simulink model "HCU_V2_Driver"  (R2023b)
settings: Solver=FixedStepAuto  StartTime=0  StopTime=2474  FixedStep=0.001  RelTol=1e-3
undefined symbols (not defined in the file or in its folder): DiscIntNeverNeededParam
libraries: autolibshared x1, slpidlib x1
settings Model: Creator=volos  LastModifiedBy=volos
settings OptimizationCC: DefaultParameterBehavior=Inlined  EnhancedBackFolding=on  PassReuseOutputArgsAs=Individual arguments  ZeroExternalMemoryAtStartup=off  ZeroInternalMemoryAtStartup=off  OptimizeBlockOrder=speed  DifferentSizesBufferReuse=on  OptimizationCustomize=off  EfficientTunableParamExpr=on
settings DebuggingCC: ParameterTunabilityLossMsg=error
settings SFSimCC: MATLABDynamicMemAlloc=off
settings RTWCC: Description=Embedded Coder  SystemTargetFile=ert.tlc  TemplateMakefile=ert_default_tmf  TargetLang=C++
settings CodeAppCC: ForceParamTrailComments=on  IgnoreCustomStorageClasses=off  OperatorAnnotations=on  SimulinkDataObjDesc=on  SFDataObjDesc=on  InsertBlockDesc=on
settings ERTTargetCC: TargetLangStandard=C++11 (ISO)  GenerateSampleERTMain=on  CodeInterfacePackaging=C++ class  InlinedParameterPlacement=NonHierarchical  RootIOFormat=Structure reference  ERTCustomFileTemplate=example_file_process.tlc

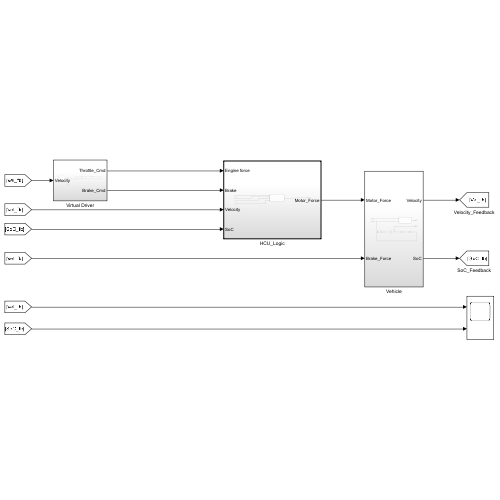
[thumbnail: Simulink's stored preview of the top-level diagram]
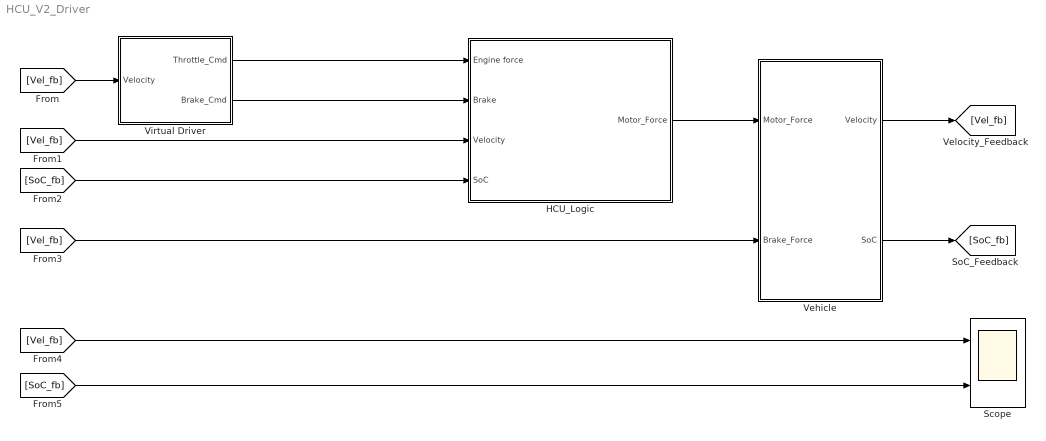
== system HCU_V2_Driver ==
  HCU_Logic : Subsystem  TreatAsAtomicUnit=on
  Scope : Scope  NumInputPorts=2
  Vehicle : Subsystem
  Virtual Driver : Subsystem
  wires:
  Virtual Driver/1(Throttle_Cmd) -> HCU_Logic/1(Engine force)
  Virtual Driver/2(Brake_Cmd) -> HCU_Logic/2(Brake)
  Vehicle/2(SoC) -> [SoC_fb]
  Vehicle/1(Velocity) -> [Vel_fb]
  HCU_Logic/1(Motor_Force) -> Vehicle/1(Motor_Force)
  [Vel_fb] -> Virtual Driver/1(Velocity)
  [Vel_fb] -> HCU_Logic/3(Velocity)
  [SoC_fb] -> HCU_Logic/4(SoC)
  [Vel_fb] -> Vehicle/2(Brake_Force)
  [Vel_fb] -> Scope/1
  [SoC_fb] -> Scope/2

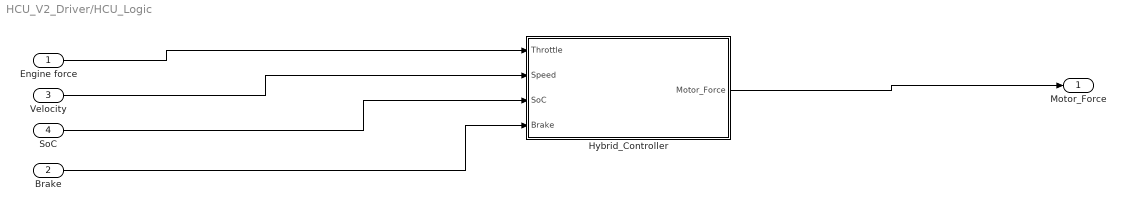
== system HCU_V2_Driver/HCU_Logic ==
  Engine force : Inport
  Brake : Inport  Port=2
  Velocity : Inport  Port=3
  SoC : Inport  Port=4
  Hybrid_Controller : Stateflow chart  TreatAsAtomicUnit=on
  Motor_Force : Outport
  wires:
  Velocity/1 -> Hybrid_Controller/2(Speed)
  Hybrid_Controller/1(Motor_Force) -> Motor_Force/1
  Engine force/1 -> Hybrid_Controller/1(Throttle)
  SoC/1 -> Hybrid_Controller/3(SoC)
  Brake/1 -> Hybrid_Controller/4(Brake)

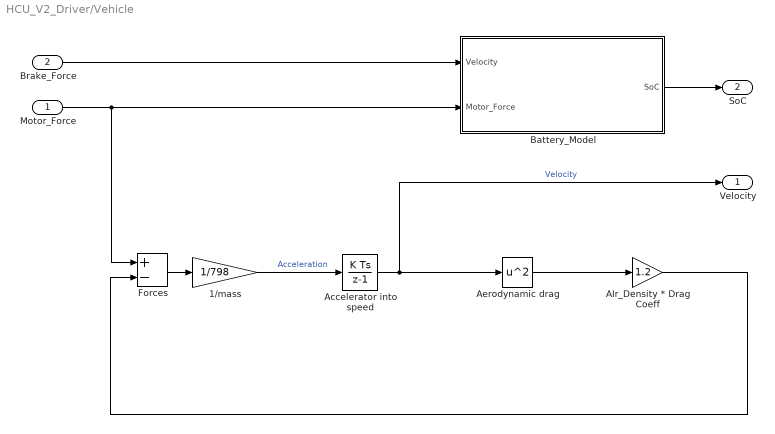
== system HCU_V2_Driver/Vehicle ==
  Motor_Force : Inport
  Brake_Force : Inport  Port=2
  1/mass : Gain  Gain=1/798
  AIr_Density * Drag Coeff : Gain  Gain=1.2
  Accelerator into speed : DiscreteIntegrator  SampleTime=-1  ICPrevOutput=DiscIntNeverNeededParam  ICPrevScaledInput=DiscIntNeverNeededParam
  Aerodynamic drag : Math  Operator=square
  Battery_Model : Subsystem
  Forces : Sum  Inputs=+-
  Velocity : Outport
  SoC : Outport  Port=2
  wires:
  Motor_Force/1 -> Battery_Model/2(Motor_Force), Forces/1
  1/mass/1 -> Accelerator into speed/1  "Acceleration"
  Aerodynamic drag/1 -> AIr_Density * Drag Coeff/1
  Brake_Force/1 -> Battery_Model/1(Velocity)
  AIr_Density * Drag Coeff/1 -> Forces/2
  Forces/1 -> 1/mass/1
  Battery_Model/1(SoC) -> SoC/1
  Accelerator into speed/1 -> Velocity/1, Aerodynamic drag/1  "Velocity"

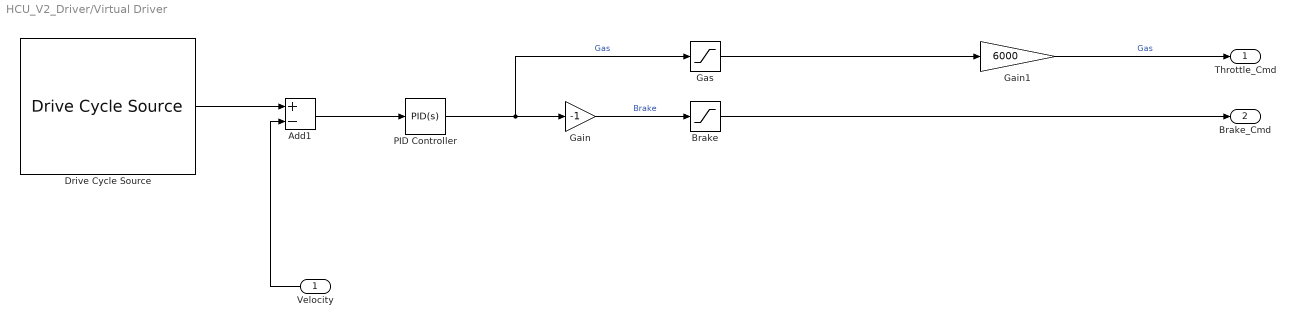
== system HCU_V2_Driver/Virtual Driver ==
  Velocity : Inport
  Add1 : Sum  Inputs=+-
  Brake : Saturate  UpperLimit=1  LowerLimit=0
  Drive Cycle Source : autolibshared/Drive Cycle Source  cycleVar=FTP75  fileVar=cycleFTP75.mat  tfinal="2474  seconds"  cycleRepeat=off  outAccPort=off  outGearPort=off  gearList=No gear data  t_wot1=5  xdot_woto=0  xdot_wot1=30  t_wot2=20  xdot_wot2=0  t_wotend=30  srcUnit=m/s  outUnit=m/s  srcAccUnit=m/s/s  outAccUnit=m/s^2  dt=0  aMode=2  faultOption=off  velBnd=2  velBndUnit=mph  inUnit=m/s  timeBnd=1  failOption=off  stopSim=off  maxFaultCnt=10  maxFaultTime=2  maxTotFaultTime=15  traceOption=off  dtTrace=1  traceWindow=10  lastDCname=FTP75  lastOutUnit=mph  lastDT=0  lastTB=1  lastSB=2  forceCalcBound=off
      settings: LibrarySourceBlock=vdynlib/Vehicle Scenarios/Drive Cycle and Maneuvers/Drive Cycle Source
  Gain : Gain  Gain=-1
  Gain1 : Gain  Gain=6000
  Gas : Saturate  UpperLimit=1  LowerLimit=0
  PID Controller : slpidlib/PID Controller  Controller=PID  Form=Parallel  TimeDomain=Continuous-time  UseExternalTs=off  SampleTime=-1  IntegratorMethod=Forward Euler  FilterMethod=Forward Euler  ControllerParametersSource=internal  P=500  I=10  UseKiTs=off  D=0  N=100  UseFilter=on  TunerSelectOption=Transfer Function Based (PID Tuner App)  InitialConditionSource=internal  InitialConditionForIntegrator=0  InitialConditionForFilter=0  DifferentiatorICPrevScaledInput=0  ExternalReset=none  TrackingMode=off  Kt=1  LimitOutput=off  SatLimitsSource=internal  UpperSaturationLimit=inf  LowerSaturationLimit=-inf  LinearizeAsGain=on  AntiWindupMode=none  Kb=1  LimitIntegrator=off  UpperIntegratorSaturationLimit=inf  LowerIntegratorSaturationLimit=-inf  POutMin=[]  POutMax=[]  IOutMin=[]  IOutMax=[]  DOutMin=[]  DOutMax=[]  NOutMin=[]  NOutMax=[]  SumOutMin=[]  SumOutMax=[]  SaturationOutMin=[]  SaturationOutMax=[]  PParamMin=[]  PParamMax=[]  IParamMin=[]  IParamMax=[]  DParamMin=[]  DParamMax=[]  NParamMin=[]  NParamMax=[]  KbParamMin=[]  KbParamMax=[]  KtParamMin=[]  KtParamMax=[]  KbOutMin=[]  KbOutMax=[]  KtOutMin=[]  KtOutMax=[]  IntegratorOutMin=[]  IntegratorOutMax=[]  FilterOutMin=[]  FilterOutMax=[]  SumI1OutMin=[]  SumI1OutMax=[]  SumI2OutMin=[]  SumI2OutMax=[]  SumI3OutMin=[]  SumI3OutMax=[]  SumI4OutMin=[]  SumI4OutMax=[]  SumDOutMin=[]  SumDOutMax=[]  DifferentiatorOutMin=[]  DifferentiatorOutMax=[]  FilterDiffOutCoefMin=[]  FilterDiffOutCoefMax=[]  ReciprocalOutMin=[]  ReciprocalOutMax=[]  SumDenOutMin=[]  SumDenOutMax=[]  SumNumOutMin=[]  SumNumOutMax=[]  DivideOutMin=[]  DivideOutMax=[]  UdiffTsProdOutMin=[]  UdiffTsProdOutMax=[]  NTsProdOutMin=[]  NTsProdOutMax=[]  UintegralTsProdOutMin=[]  UintegralTsProdOutMax=[]  UngainTsProdOutMin=[]  UngainTsProdOutMax=[]  ClampingZeroOutDataTypeStr=Inherit: Inherit via back propagation  ClampingZeroOutMin=[]  ClampingZeroOutMax=[]  FilterDenConstantOutDataTypeStr=Inherit: Inherit via back propagation  FilterDenConstantOutMin=[]  FilterDenConstantOutMax=[]  PCopyOutDataTypeStr=Inherit: Inherit via back propagation  PCopyOutMin=[]  PCopyOutMax=[]  NCopyOutDataTypeStr=Inherit: Inherit via back propagation  NCopyOutMin=[]  NCopyOutMax=[]  IntegratorContinuousStateAttributes=''  IntegratorStateMustResolveToSignalObject=off  IntegratorRTWStateStorageClass=Auto  FilterContinuousStateAttributes=''  FilterStateMustResolveToSignalObject=off  FilterRTWStateStorageClass=Auto  ParallelPVariant=InternalParameters  IdealPVariant=Disabled  IVariant=InternalParameters  DVariant=InternalParameters  IntegratorVariant=Continuous  SatVariant=Disabled  AWVariant=Passthrough  PCopyVariant=Disabled  TRVariant=Disabled  FdbkBlocksVariant=Forward  IdealPFdbkVariant=Disabled  SatFdbkVariant=Disabled  DerivativeFilterVariant=ContFilter  NVariant=InternalParameters  NCopyVariant=Disabled  FilterICVariant=InternalICsFilter  IntegratorICVariant=InternalICs  ExternalResetVariant=Disabled  TRSumVariant=Passthrough  SumFdbkVariant=Disabled  SumVariant=Sum_PID  TsampFilterVariant=InternalTs  TsampNgainVariant=Passthrough  TsampIntegralVariant=Disabled_SignalSpec  ExternalSaturationOutDataTypeStr=Inherit: Same as second input
  Throttle_Cmd : Outport
  Brake_Cmd : Outport  Port=2
  wires:
  Gain1/1 -> Throttle_Cmd/1  "Gas"
  Velocity/1 -> Add1/2
  Gas/1 -> Gain1/1
  Gain/1 -> Brake/1  "Brake"
  Drive Cycle Source/1 -> Add1/1
  PID Controller/1 -> Gas/1, Gain/1  "Gas"
  Add1/1 -> PID Controller/1
  Brake/1 -> Brake_Cmd/1

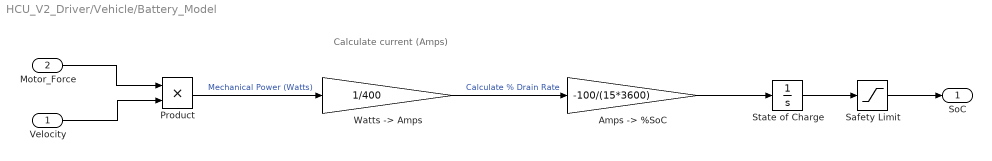
== system HCU_V2_Driver/Vehicle/Battery_Model ==
  note: Calculate current (Amps)
  Velocity : Inport
  Motor_Force : Inport  Port=2
  "Amps -> %SoC" : Gain  Gain=-100/(15*3600)
  Product : Product
  Safety Limit : Saturate  UpperLimit=100  LowerLimit=0
  State of Charge : Integrator  InitialCondition=90
  "Watts -> Amps" : Gain  Gain=1/400
  SoC : Outport
  wires:
  Motor_Force/1 -> Product/1
  Velocity/1 -> Product/2
  Product/1 -> "Watts -> Amps"/1  "Mechanical Power (Watts)"
  "Watts -> Amps"/1 -> "Amps -> %SoC"/1  "Calculate % Drain Rate"
  "Amps -> %SoC"/1 -> State of Charge/1
  State of Charge/1 -> Safety Limit/1
  Safety Limit/1 -> SoC/1

== stateflow chart HCU_V2_Driver/HCU_Logic/Hybrid_Controller ==
  state Battery_Regen_Mode
    entry:
    Motor_Force=-4000;
  note: Motor is pushing backwards/slowing down
  state Eco_mode
    entry:
    Motor_Force=0;
  state Boost_Mode
    entry:
    Motor_Force = 3000;
  note: When in Boost Mode, add 3000N of electric thrust
  note: When in Eco Mode, electric motor is OFF
  Eco_mode -> Battery_Regen_Mode [order 2] : [Brake > 0]
  Boost_Mode -> Battery_Regen_Mode [order 2] : [Brake > 0]
  Battery_Regen_Mode -> Eco_mode : [Brake == 0]
  (default) -> Eco_mode
  Eco_mode -> Boost_Mode [order 1] : [Throttle >= 5500 && SoC >20]
  Boost_Mode -> Eco_mode [order 1] : [Throttle < 5500]
  data: Throttle input; Speed input; Motor_Force output; SoC input; Brake input
